simulink model "simulink2CRRCSim"  (Simulink 7.9)
settings: Solver=ode45  StartTime=0.0  StopTime=inf  RelTol=1e-3
libraries: aerolibanimutils x1, dspnetwork x1
settings Model: Creator=jan  LastModifiedBy=jan

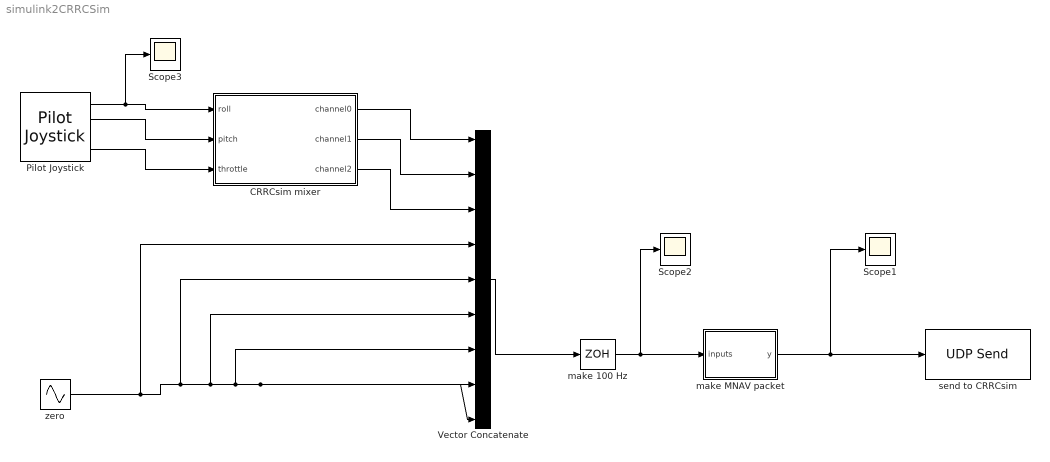
== system simulink2CRRCSim ==
  CRRCsim mixer : MATLAB Function  TreatAsAtomicUnit=on
  Pilot Joystick : aerolibanimutils/Pilot Joystick  JoystickID=Joystick1  OutputConfiguration=FourAxis  SampleTime=1/30
  Scope1 : Scope
      settings: YMin=0  YMax=70000
  Scope2 : Scope
  Scope3 : Scope
      settings: SaveName=ScopeData2
  Vector Concatenate : Concatenate  NumInputs=9
  make 100 Hz : ZeroOrderHold  SampleTime=0.01
  make MNAV packet : MATLAB Function  TreatAsAtomicUnit=on
  send to CRRCsim : dspnetwork/UDP Send  remoteURL='127.0.0.1'  remotePort=9002  localURL='0.0.0.0'  localPortSource=Automatically determine  localPort=-1  sampletime=-1  separateLengthPort=0
  zero : Sin  Amplitude=0  SampleTime=0
  wires:
  make 100 Hz/1 -> make MNAV packet/1(inputs), Scope2/1
  Vector Concatenate/1 -> make 100 Hz/1
  make MNAV packet/1(y) -> send to CRRCsim/1, Scope1/1
  zero/1 -> Vector Concatenate/7, Vector Concatenate/9, Vector Concatenate/8, Vector Concatenate/6, Vector Concatenate/5, Vector Concatenate/4
  Pilot Joystick/1 -> CRRCsim mixer/1(roll), Scope3/1
  Pilot Joystick/2 -> CRRCsim mixer/2(pitch)
  Pilot Joystick/4 -> CRRCsim mixer/3(throttle)
  CRRCsim mixer/1(channel0) -> Vector Concatenate/1
  CRRCsim mixer/2(channel1) -> Vector Concatenate/2
  CRRCsim mixer/3(channel2) -> Vector Concatenate/3

== matlab function CRRCsim mixer ==
  data: roll input double; channel0 output double; pitch input double; throttle input double; channel1 output double; channel2 output double
% Takes roll, pitch, throttle as inputs and maps
% it to the appropriate channels to send it to
% the MNAV interface of CRRCSim
function [channel0,channel1,channel2] =  CRRCSimMixer(roll, pitch, throttle)
%#codegen
channel2 = throttle;

end

== matlab function make MNAV packet ==
  data: inputs input double; y output double
% Takes an input argument and turns it into 9 equal servo
% commands packed into a MNAV protocol message.
% Input is a vector of 9 double [-1, 1].
function y =  makeMNAV(inputs)
%#codegen
% Create bytes of message:
startByte1= uint8('U');
startByte2= uint8('U');
messageIDByte1= uint8('S');
messageIDByte2= uint8('S');
servobyte32Bit1 = zeros(9,1,'uint32');
servobyte32Bit2 = zeros(9,1,'uint32');
servo32Bit = zeros(9,1,'uint32');

checksum = uint32(0);
checksum = uint32(messageIDByte1) + uint32(messageIDByte2);
for i=1:9
    servo32Bit(i) = uint32(32767 + inputs(i)*32000);
    servoBytes = typecast(servo32Bit(i), 'uint8');
    servobyte32Bit1(i) = uint32(servoBytes(1));
    servobyte32Bit2(i) = uint32(servoBytes(2));
    checksum = checksum + servobyte32Bit1(i) + servobyte32Bit2(i);
end

checksumBytes = typecast(checksum, 'uint8');

message = zeros(6+18, 1, 'uint8');
message(1,1) = startByte1;
message(2,1) = startByte2;
message(3,1) = messageIDByte1;
message(4,1) = messageIDByte2;
channelIndex = 1;
for i=1:2:18
    servoValueinBytes = typecast(servo32Bit(channelIndex), 'uint8');
    message(4+i,1) = servoValueinBytes(2);
    message(4+i+1,1) = servoValueinBytes(1);
    channelIndex = channelIndex + 1;
end
message(23,1) = checksumBytes(2);
message(24,1) = checksumBytes(1);

y = message;
end
